simulink model "s0520"  (Simulink 7.0)
settings: Solver=ode3  SolverMode=SingleTasking  StartTime=0.0  StopTime=900  FixedStep=1  MaxStep=1  RelTol=1e-3  AbsTol=1e-6
values from neighbouring files (symbols this model uses):
  Kpr = 10    [m0108d.m]    (also in m0109b.m = 1; m0113c.m; m0404Bsp.m = 3)
  schalt = 3    [m0314.m]    (also in m0319.m; m0322.m)
  T1 = 3*T1    (= 0.3)    [m0203.m]    (also in m0204.m = 0.1; m0205.m = 0.1; m0207.m = 0.1; m0221d.m = 1/a0)
  Tt = .4    (= 0.4)    [m0108d.m]    (also in m0259.m = 1; m0314.m = 2.13; m0322.m = 0.8; m0326.m = 4)
  wdach = 0    [m0109b.m]    (also in m0404Bsp.m = 1)
undefined symbols (not defined in the file or in its folder): snen, szae, Tn, Tv
settings Model: Creator=froriep  LastModifiedBy=froriep
settings DataIOCC: LimitDataPoints=off  SaveOutput=off  TimeSaveName=t
settings OptimizationCC: BooleanDataType=off  InlineInvariantSignals=on
settings DebuggingCC: SaveWithParameterizedLinksMsg=none  SignalResolutionControl=TryResolveAllWithWarning  SolverPrmCheckMsg=none  MultiTaskDSMMsg=warning  MultiTaskCondExecSysMsg=none  StrictBusMsg=None
settings HardwareCC: TargetUnknown=on
settings RTWCC: IncludeERTFirstTime=on
settings GRTTargetCC: TargetFcnLib=ansi_tfl_tmw.mat  ModelReferenceCompliant=off  CompOptLevelCompliant=off  MatFileLogging=off

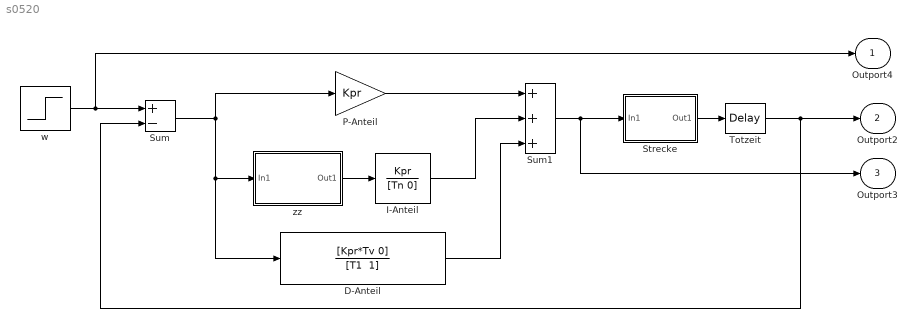
== system s0520 ==
  D-Anteil : TransferFcn  Numerator=[Kpr*Tv 0]  Denominator="[T1  1]"
  I-Anteil : TransferFcn  Numerator=Kpr  Denominator=[Tn 0]
  P-Anteil : Gain  Gain=Kpr  ParameterDataType=sfix(16)  ParameterScaling=2^0  OutDataType=sfix(16)  OutScaling=2^0  SaturateOnIntegerOverflow=on
  Strecke : Subsystem
      mask Display: disp('Gs(s)')
  Sum : Sum  Inputs=+-  OutDataType=sfix(16)  OutScaling=2^0  SaturateOnIntegerOverflow=on  InputSameDT=on
  Sum1 : Sum  Inputs=+++  OutDataType=sfix(16)  OutScaling=2^0  SaturateOnIntegerOverflow=on  InputSameDT=on
  Totzeit : TransportDelay  DelayTime=Tt
  w : Step  Time=0  After=wdach  SampleTime=0
  zz : Subsystem
      mask Display: disp('Schalter')
  Outport4 : Outport  OutDataType=sfix(16)  OutScaling=2^0
  Outport2 : Outport  Port=2  OutDataType=sfix(16)  OutScaling=2^0
  Outport3 : Outport  Port=3  OutDataType=sfix(16)  OutScaling=2^0
  wires:
  I-Anteil/1 -> Sum1/2
  zz/1(Out1) -> I-Anteil/1
  Totzeit/1 -> Sum/2, Outport2/1
  Strecke/1(Out1) -> Totzeit/1
  w/1 -> Outport4/1, Sum/1
  D-Anteil/1 -> Sum1/3
  Sum/1 -> P-Anteil/1, D-Anteil/1, zz/1(In1)
  P-Anteil/1 -> Sum1/1
  Sum1/1 -> Outport3/1, Strecke/1(In1)

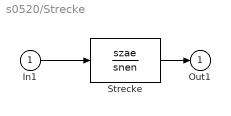
== system s0520/Strecke ==
  In1 : Inport  OutDataType=sfix(16)  OutScaling=2^0
  Strecke : TransferFcn  Numerator=szae  Denominator=snen
  Out1 : Outport  OutDataType=sfix(16)  OutScaling=2^0
  wires:
  In1/1 -> Strecke/1
  Strecke/1 -> Out1/1

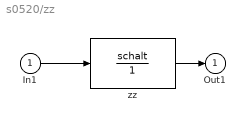
== system s0520/zz ==
  In1 : Inport  OutDataType=sfix(16)  OutScaling=2^0
  zz : TransferFcn  Numerator=schalt  Denominator=1
  Out1 : Outport  OutDataType=sfix(16)  OutScaling=2^0
  wires:
  In1/1 -> zz/1
  zz/1 -> Out1/1
